simulink model "ball_beam_closedloop"  (R2024a)
settings: Solver=VariableStepAuto  StartTime=0.0  StopTime=10.0  RelTol=1e-3
undefined symbols (not defined in the file): Kp_tuned, Td
libraries: simulink x1
settings Model: Creator=jorda  LastModifiedBy=jorda

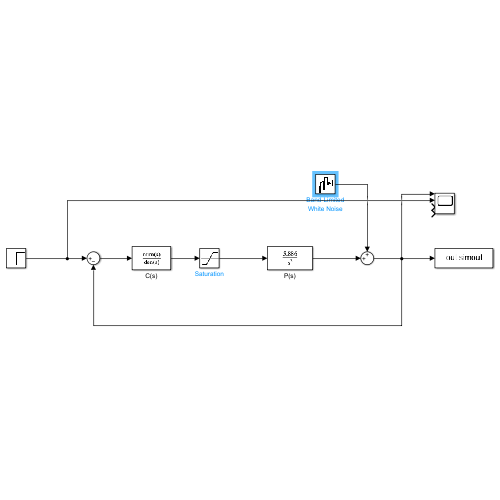
[thumbnail: Simulink's stored preview of the top-level diagram]
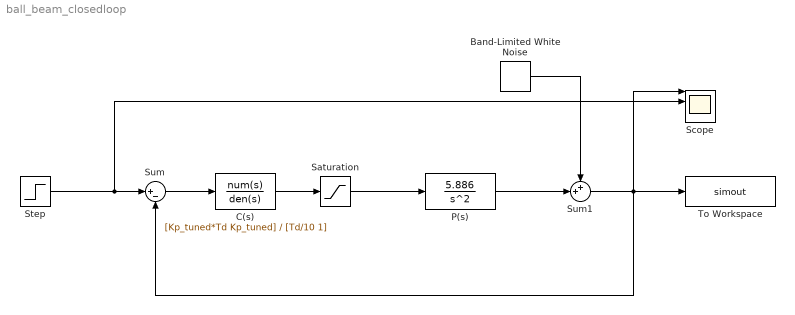
== system ball_beam_closedloop ==
  Band-Limited White Noise : simulink/Sources/Band-Limited White Noise  Cov=[1e-7]  Ts=0.1  seed=[23341]
  C(s) : TransferFcn  Numerator=[Kp_tuned*Td Kp_tuned]  Denominator=[Td/10 1]
  P(s) : TransferFcn  Numerator=[5.886]  Denominator=[1 0 0]
  Saturation : Saturate  UpperLimit=0.2618  LowerLimit=-0.2618
  Scope : Scope  NumInputPorts=4
  Step : Step  After=0.15  SampleTime=0
  Sum : Sum  Inputs=|+-
  Sum1 : Sum  Inputs=++|
  To Workspace : ToWorkspace  VariableName=simout  SaveFormat=Timeseries  SampleTime=-1
  wires:
  Sum1/1 -> Scope/1, Sum/2, To Workspace/1
  Band-Limited White Noise/1 -> Sum1/1
  Saturation/1 -> P(s)/1
  P(s)/1 -> Sum1/2
  C(s)/1 -> Saturation/1
  Sum/1 -> C(s)/1
  Step/1 -> Scope/2, Sum/1
